simulink model "ropestop_cal"  (R2023a)
settings: Solver=VariableStepAuto  StartTime=0.0  StopTime=5  RelTol=1e-3
values from neighbouring files (symbols this model uses):
  L = 50.0    [data.sldd]    (also in k_cal.m = getValue(getEntry(sectionObj, 'L')))
settings Model: DataDictionary=data.sldd  Creator=MangoJuice  LastModifiedBy=MangoJuice
settings DataIOCC: SignalLogging=off  DSMLogging=off  ReturnWorkspaceOutputs=off
settings RTWCC: GPUComputeCapability=5.0
settings ConfigComp: CovBoundaryAbsTol=1.0e-5

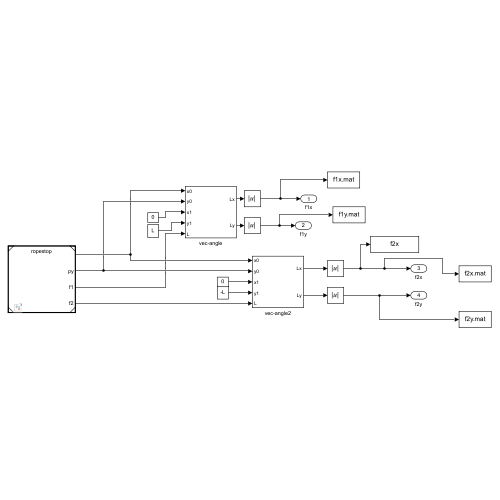
[thumbnail: Simulink's stored preview of the top-level diagram]
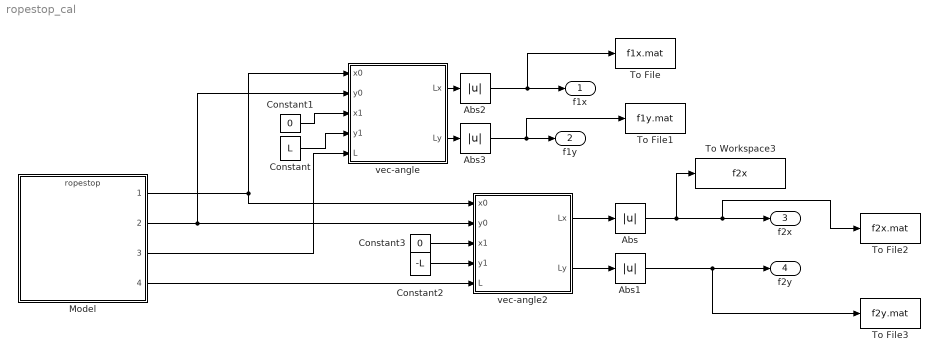
== system ropestop_cal ==
  Abs{,1..3} (4 alike) : Abs  SaturateOnIntegerOverflow=off
  Constant : Constant  Value=L
  Constant1 : Constant  Value=0
  Constant2 : Constant  Value=-L
  Constant3 : Constant  Value=0
  Model : ModelReference  ModelNameDialog=ropestop.slx  SimulationMode=Normal  ModelReferenceVersion=1.19
  To File : ToFile  Filename=f1x.mat  MatrixName=f1x  SaveFormat=Timeseries
  To File1 : ToFile  Filename=f1y.mat  MatrixName=f1y  SaveFormat=Timeseries
  To File2 : ToFile  Filename=f2x.mat  MatrixName=f2x  SaveFormat=Timeseries
  To File3 : ToFile  Filename=f2y.mat  MatrixName=f2y  SaveFormat=Timeseries
  To Workspace3 : ToWorkspace  VariableName=f2x  SaveFormat=Timeseries  SampleTime=-1
  vec-angle : Subsystem
  vec-angle2 : Subsystem
  f1x : Outport
  f1y : Outport  Port=2
  f2x : Outport  Port=3
  f2y : Outport  Port=4
  wires:
  Model/1 -> vec-angle2/1(x0), vec-angle/1(x0)
  Model/2 -> vec-angle2/2(y0), vec-angle/2(y0)
  Constant1/1 -> vec-angle/3(x1)
  Constant/1 -> vec-angle/4(y1)
  Constant2/1 -> vec-angle2/4(y1)
  Constant3/1 -> vec-angle2/3(x1)
  Model/3 -> vec-angle/5(L)
  vec-angle/2(Ly) -> Abs3/1
  Model/4 -> vec-angle2/5(L)
  vec-angle2/1(Lx) -> Abs/1
  vec-angle2/2(Ly) -> Abs1/1
  Abs1/1 -> To File3/1, f2y/1
  Abs/1 -> To Workspace3/1, To File2/1, f2x/1
  vec-angle/1(Lx) -> Abs2/1
  Abs2/1 -> To File/1, f1x/1
  Abs3/1 -> To File1/1, f1y/1

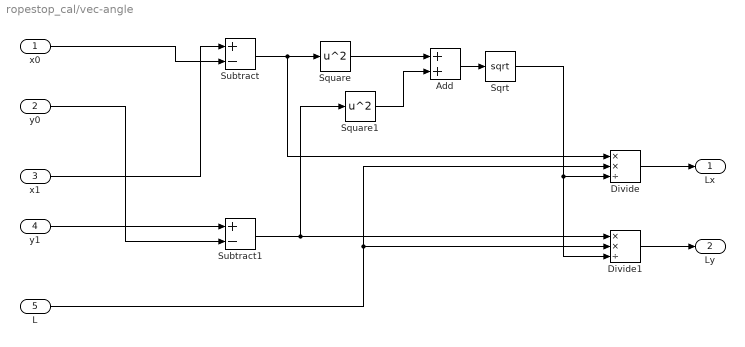
== system ropestop_cal/vec-angle ==
  x0 : Inport
  y0 : Inport  Port=2
  x1 : Inport  Port=3
  y1 : Inport  Port=4
  L : Inport  Port=5
  Add : Sum
  Divide : Product  Inputs=**/
  Divide1 : Product  Inputs=**/
  Sqrt : Sqrt
  Square : Math  Operator=square
  Square1 : Math  Operator=square
  Subtract : Sum  Inputs=+-
  Subtract1 : Sum  Inputs=+-
  Lx : Outport
  Ly : Outport  Port=2
  wires:
  x0/1 -> Subtract/2
  x1/1 -> Subtract/1
  y1/1 -> Subtract1/1
  y0/1 -> Subtract1/2
  Subtract1/1 -> Divide1/1, Square1/1
  Subtract/1 -> Divide/1, Square/1
  Square/1 -> Add/1
  Square1/1 -> Add/2
  Add/1 -> Sqrt/1
  L/1 -> Divide1/2, Divide/2
  Sqrt/1 -> Divide1/3, Divide/3
  Divide/1 -> Lx/1
  Divide1/1 -> Ly/1

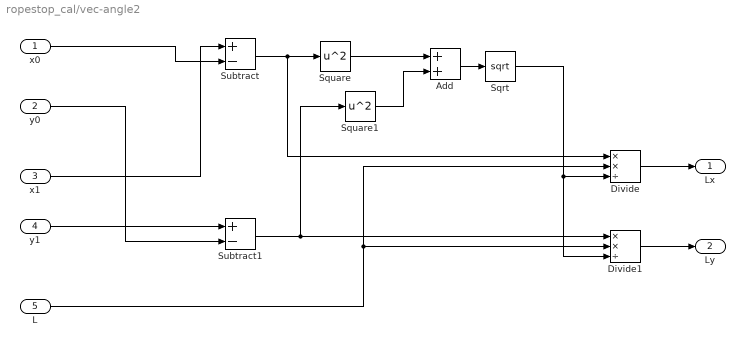
== system ropestop_cal/vec-angle2 ==
  x0 : Inport
  y0 : Inport  Port=2
  x1 : Inport  Port=3
  y1 : Inport  Port=4
  L : Inport  Port=5
  Add : Sum
  Divide : Product  Inputs=**/
  Divide1 : Product  Inputs=**/
  Sqrt : Sqrt
  Square : Math  Operator=square
  Square1 : Math  Operator=square
  Subtract : Sum  Inputs=+-
  Subtract1 : Sum  Inputs=+-
  Lx : Outport
  Ly : Outport  Port=2
  wires:
  Divide1/1 -> Ly/1
  Divide/1 -> Lx/1
  Sqrt/1 -> Divide/3, Divide1/3
  L/1 -> Divide/2, Divide1/2
  Add/1 -> Sqrt/1
  Square1/1 -> Add/2
  Square/1 -> Add/1
  Subtract/1 -> Square/1, Divide/1
  Subtract1/1 -> Square1/1, Divide1/1
  y0/1 -> Subtract1/2
  y1/1 -> Subtract1/1
  x1/1 -> Subtract/1
  x0/1 -> Subtract/2
